simulink model "ImpulseModelOnly"  (R2012b)
settings: Solver=ode45  StartTime=0.0  StopTime=10  RelTol=1e-3
settings Model: Creator=kyle  LastModifiedBy=kyle
settings DataIOCC: InspectSignalLogs=on

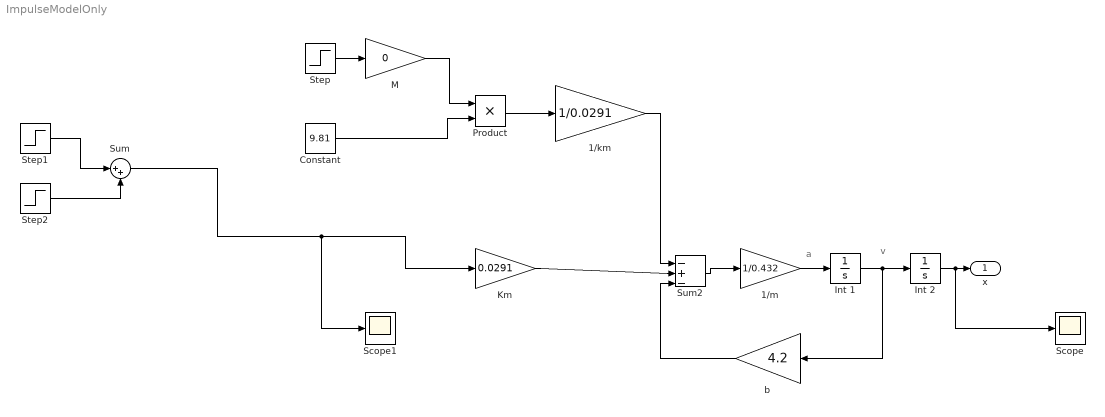
== system ImpulseModelOnly ==
  note: a
  note: v
  1/km : Gain  Gain=1/0.0291
  1/m : Gain  Gain=1/0.432
  Constant : Constant  Value=9.81
  Int 1 : Integrator
  Int 2 : Integrator
  Km : Gain  Gain=0.0291
  M : Gain  Gain=0
  Product : Product  RndMeth=Zero
  Scope : Scope
  Scope1 : Scope
  Step : Step  SampleTime=0
  Step1 : Step  Time=.1  After=-100  SampleTime=0
  Step2 : Step  Time=0  After=100  SampleTime=0
  Sum : Sum  Inputs=|++
  Sum2 : Sum  Inputs=|-+-
  b : Gain  Gain=4.2
  x : Outport
  wires:
  Km/1 -> Sum2/2
  b/1 -> Sum2/3
  Sum2/1 -> 1/m/1
  Int 1/1 -> Int 2/1, b/1
  Int 2/1 -> Scope/1, x/1
  1/km/1 -> Sum2/1
  1/m/1 -> Int 1/1
  Constant/1 -> Product/2
  M/1 -> Product/1
  Product/1 -> 1/km/1
  Step/1 -> M/1
  Step1/1 -> Sum/1
  Step2/1 -> Sum/2
  Sum/1 -> Scope1/1, Km/1
